simulink model "vehicle_model_2025"  (R2025a)
settings: Solver=ode23tb  StartTime=0.0  StopTime=20  MaxStep=0.001  RelTol=1e-3
model workspace (MAT data in the model file):
  init_r = 0
  init_vx = 0
  init_vy = 0
values from neighbouring files (symbols this model uses):
  Par =     [0_Load_data.mat]
  TireData =     [0_Load_data.mat]
undefined symbols (not defined in the file or in its folder): aero_par, Battery, Motor, SimInput_Steer, SimInput_TorqueFL, SimInput_TorqueFR, SimInput_TorqueRL, SimInput_TorqueRR, sus_par
libraries: simulink x4, BatteryEstimators x1
(part 2 of 2)

== matlab function vehicle_model_2025/Camber/MATLAB Function ==
  data: gamma_FR output; ay input; gamma_FL output; gamma_RL output; gamma_RR output; delta input; Par parameter; sus_par parameter
function [gamma_FR,gamma_FL,gamma_RL,gamma_RR] = fcn(ay,delta,Par, sus_par)

%% Static camber
gamma_static = sus_par.Camber_static;
% track_width = par.TW;
%% SUSPENSION ROLL STIFFNESS
k_phi1 = 10014;  % front axle roll stiffness (Nm/rad)
k_phi2 = 11466;  % rear axle roll stiffness (Nm/rad)

%% ROLL CENTER HEIGHTS
q1 = 0.062;      % front roll center height (m)
q2 = 0.091;      % rear roll center height (m)

%% CAMBER GEOMETRY
b1 = 0.20;       % front IC horizontal distance (m)
b2 = 0.22;       % rear IC horizontal distance (m)

%% TOTAL ROLL STIFFNESS
k_phi_total = k_phi1 + k_phi2;

%% TOTAL VEHICLE ROLL ANGLE
phi = Par.m.*ay.*Par.CG_h / k_phi_total;   % rad

%% AXLE ROLL ANGLES
phi_s1 = phi * (k_phi1 / k_phi_total);   % front suspension roll
phi_s2 = phi * (k_phi2 / k_phi_total);   % rear suspension roll

% Zwc_f = track_width.*0.5.*phi_s1;
% Zwc_r = track_width.*0.5.*phi_s2;
%% CAMBER GAIN COEFFICIENTS
k_gamma_f = - (q1 - b1) / b1;   % front
k_gamma_r = - (q2 - b2) / b2;   % rear

%% Camber due to roll on front axle
delta_gamma_roll_f = k_gamma_f * phi_s1;

%% Camber due to roll on rear axle
delta_gamma_roll_r = k_gamma_r * phi_s2;

%% Camber gain due to heave
% delta_gamma_heave_f = atan(Zwc_f/par.L_fvsa);
% delta_gamma_heave_r = atan(Zwc_r/par.L_fvsa);

%% Camber due to caster 
delta_gamma_caster = atan(tan(sus_par.Caster_static).*sin(delta));

%% Camber angle
gamma_FL = gamma_static + delta_gamma_roll_f + delta_gamma_caster;
gamma_FR = gamma_static - (delta_gamma_roll_f + delta_gamma_caster);
gamma_RL = gamma_static + delta_gamma_roll_r + delta_gamma_caster;
gamma_RR = gamma_static - (delta_gamma_roll_r + delta_gamma_caster);

== matlab function vehicle_model_2025/Simplified Tire Model ==
  data: Fz input; Fx output size=4; slip_ratios input; slip_angles input; camber_angles input; Fy output size=4; Mz output size=4; Mu_x output size=4; Mu_y output size=4; TireData parameter; Par parameter; sus_par parameter
function [Fx, Fy, Mz, Mu_x, Mu_y] = fcn(Fz, slip_ratios, slip_angles, camber_angles, TireData,Par,sus_par)
%#codegen
% =========================================================================
%  VECTORIZED MAGIC FORMULA 5.2 (4-WHEEL)
%  Computes tire physics for all 4 corners simultaneously using element-wise math.
%
%  INPUTS (All 4x1 Vectors):
%    Fz    : Vertical Loads [N] -> [FL; FR; RL; RR]
%    Kappa : Slip Ratios [-]
%    Alpha : Slip Angles [rad]
%    Gamma : Camber Angles [rad]
%    TireData : Parameter Struct (Must be loaded in Base Workspace)
%
%  OUTPUTS (All 4x1 Vectors):
%    Fx    : Longitudinal Force [N]
%    Fy    : Lateral Force [N]
%    Mz    : Self-Aligning Torque [Nm]
%    Mu_x  : Long. Friction Coeff [-]
%    Mu_y  : Lat. Friction Coeff [-]
% =========================================================================

    % 1. EXTRACT PARAMETERS (Scalars)
    p = TireData;
    s = TireData.Scales;
    Fz0 = p.FNOMIN;
    R0  = p.R0;
    par = Par;
    % 2. INPUT SAFETY & NORMALIZATION
    % Clamp negative loads to 0 (Tires can't pull ground)
    Fz_safe = max(Fz, 0); 
    
    % Avoid division by zero for Mu calculations later
    Fz_denom = max(Fz_safe, 1.0); 

    % Normalized Load (dfz) - Vectorized
    dfz = (Fz_safe - Fz0) ./ Fz0;

    % ---------------------------------------------------------------------
    % A. LONGITUDINAL FORCE (Fx) - VECTORIZED
    % ---------------------------------------------------------------------
    Cx = p.PCX1 * s.LCX;
    
    % Friction Coeff Mu_x
    mu_x_base = (p.PDX1 + p.PDX2 .* dfz) .* (1 - p.PDX3 .* camber_angles.^2) .* s.LMUX;
    Dx = mu_x_base .* Fz_safe;
    
    % Stiffness Kx
    Kx = Fz_safe .* (p.PKX1 + p.PKX2 .* dfz) .* exp(p.PKX3 .* dfz) .* s.LKX;
    
    % Stiffness Factor Bx
    Bx = Kx ./ (Cx .* Dx + 1e-6); 
    
    % Shifts (Horizontal & Vertical)
    Shx = (p.PHX1 + p.PHX2 .* dfz) .* s.LHX;
    Svx = Fz_safe .* (p.PVX1 + p.PVX2 .* dfz) .* s.LVX;
    
    % Composite Slip
    k_s = slip_ratios + Shx;
    
    % Curvature Ex (Sign Dependent)
    Ex = (p.PEX1 + p.PEX2 .* dfz + p.PEX3 .* dfz.^2) .* (1 - p.PEX4 .* sign(k_s)) .* s.LEX;
    Ex(Ex > 1) = 1; % Clamp
    
    % Calculation
    Bx_k = Bx .* k_s;
    Fx = Dx .* sin(Cx .* atan(Bx_k - Ex .* (Bx_k - atan(Bx_k)))) + Svx;

    % ---------------------------------------------------------------------
    % B. LATERAL FORCE (Fy) - VECTORIZED
    % ---------------------------------------------------------------------
    Cy = p.PCY1 * s.LCY;
    
    % Friction Coeff Mu_y
    mu_y_base = (p.PDY1 + p.PDY2 .* dfz) .* (1 - p.PDY3 .* camber_angles.^2) .* s.LMUY;
    Dy = mu_y_base .* Fz_safe;
    
    % Cornering Stiffness Ky (Trig Form)
    Ky = p.PKY1 .* Fz0 .* sin(2 .* atan(Fz_safe ./ (p.PKY2 .* Fz0))) .* (1 - p.PKY3 .* abs(camber_angles)) .* s.LKY;
    
    % Poly fallback check (if PKY2 implies poly form)
    if (Ky(1) < 1)
        Ky = Fz_safe .* (p.PKY1 + p.PKY2 .* dfz) .* s.LKY;
    end
    
    By = Ky ./ (Cy .* Dy + 1e-6);
    
    % Shifts
    Shy = (p.PHY1 + p.PHY2 .* dfz) .* s.LHY;
    Svy = Fz_safe .* (p.PVY1 + p.PVY2 .* dfz) .* s.LVY;
    
    a_s = slip_angles + 0*Shy;
    
    % Curvature Ey (Sign Dependent)
    Ey = (p.PEY1 + p.PEY2 .* dfz) .* (1 - (p.PEY3 + p.PEY4 .* camber_angles) .* sign(a_s)) .* s.LEY;
    Ey(Ey > 1) = 1;
    
    % Calculation
    By_a = By .* a_s;
    Fy = -(Dy .* sin(Cy .* atan(By_a - Ey .* (By_a - atan(By_a)))) + 0*Svy);

    % ---------------------------------------------------------------------
    % C. SELF-ALIGNING TORQUE (Mz) - VECTORIZED
    % ---------------------------------------------------------------------
    % Peak Trail Dt
    Dt = (p.QDZ1 + p.QDZ2 .* dfz) .* (1 - p.QDZ3 .* abs(camber_angles)) .* R0 .* s.LTR;
    
    % Trail Slope Bt
    Bt = (p.QBZ1 + p.QBZ2 .* dfz + p.QBZ3 .* dfz.^2) .* (1 + p.QBZ4 .* abs(camber_angles)) .* (s.LKY / s.LMUY);
    
    Ct = p.QCZ1; % Scalar
    Et = (p.QEZ1 + p.QEZ2 .* dfz + p.QEZ3 .* dfz.^2);
    
    % Trail 't' Calculation(Pneumatic trail)
    Bt_a = Bt .* a_s;
    alpha_t = Bt_a - Et .* (Bt_a - atan(Bt_a));
    t = Dt .* cos(Ct .* atan(alpha_t)) .* cos(a_s);

    % Trail 'tm' Calculation(mechanical trail)
    tm = par.R0.*tan(sus_par.Caster_static);

    % Residual Mzr
    Dr = Fz_safe .* R0 .* (p.QDZ6 + p.QDZ7 .* dfz) .* s.LRES;
    Br = 10;
    Mzr = Dr .* cos(atan(Br .* a_s));
    
    % Final Mz (Standard Restoring: Negative Slope)
    % Note: If you want positive slope (sharp tune from before), multiply term by -1.
    Mz = -(t+tm).*Fy + Mzr;

    % ---------------------------------------------------------------------
    % D. OUTPUTS (Zero out lifted wheels)
    % ---------------------------------------------------------------------
    % Friction Coeffs
    Mu_x = Fx ./ Fz_denom;
    Mu_y = Fy ./ Fz_denom;

    % Clean up lifted wheels (Fz <= 0)
    % lifted_idx = Fz <= 0;
    % Fx(lifted_idx) = 0;
    % Fy(lifted_idx) = 0;
    % Mz(lifted_idx) = 0;
    % Mu_x(lifted_idx) = 0;
    % Mu_y(lifted_idx) = 0;

end

== matlab function vehicle_model_2025/roll and pitch angles/theta_constants ==
  data: K_theta output; C_theta output; sus_par parameter; Par parameter
function [K_theta,C_theta] = fcn(sus_par,Par)

% Calculating Pitching stiffness
Kw_fl = sus_par.Ks_f.*(sus_par.Motion_ratio_f)^2; 
Kw_fr = sus_par.Ks_f.*(sus_par.Motion_ratio_f)^2;
Kw_rl = sus_par.Ks_r.*(sus_par.Motion_ratio_r)^2;
Kw_rr = sus_par.Ks_r.*(sus_par.Motion_ratio_r)^2;

K_theta = (Kw_fl + Kw_fr).*(Par.Lf)^2 + (Kw_rl + Kw_rr).*(Par.Lr)^2;

% Calculating Pitch Damping
Cw_fl = sus_par.C_damp_f.*(sus_par.Motion_ratio_f)^2;
Cw_fr = sus_par.C_damp_f.*(sus_par.Motion_ratio_f)^2;
Cw_rl = sus_par.C_damp_r.*(sus_par.Motion_ratio_r)^2;
Cw_rr = sus_par.C_damp_r.*(sus_par.Motion_ratio_r)^2;

C_theta = (Cw_fl + Cw_fr).*(Par.Lf)^2 + (Cw_rl + Cw_rr).*(Par.Lr)^2;

% Kw = [Kw_fl;Kw_fr;Kw_rl;Kw_rr];

== matlab function vehicle_model_2025/roll and pitch angles/Phi_constants ==
  data: K_phi output; C_phi output; Par parameter; sus_par parameter
function [K_phi,C_phi] = fcn(Par, sus_par)

% Calculating Pitching stiffness
Kw_fl = sus_par.Ks_f.*(sus_par.Motion_ratio_f)^2; 
Kw_fr = sus_par.Ks_f.*(sus_par.Motion_ratio_f)^2;
Kw_rl = sus_par.Ks_r.*(sus_par.Motion_ratio_r)^2;
Kw_rr = sus_par.Ks_r.*(sus_par.Motion_ratio_r)^2;

K_phi = (Kw_fl + Kw_fr).*(Par.TW/2)^2 + (Kw_rl + Kw_rr).*(Par.TW/2)^2;

% Calculating Pitch Damping
Cw_fl = sus_par.C_damp_f.*(sus_par.Motion_ratio_f)^2;
Cw_fr = sus_par.C_damp_f.*(sus_par.Motion_ratio_f)^2;
Cw_rl = sus_par.C_damp_r.*(sus_par.Motion_ratio_r)^2;
Cw_rr = sus_par.C_damp_r.*(sus_par.Motion_ratio_r)^2;

C_phi = (Cw_fl + Cw_fr).*(Par.TW/2)^2 + (Cw_rl + Cw_rr).*(Par.TW/2)^2;

== matlab function vehicle_model_2025/Battery Pack/MATLAB Function ==
  data: Voc_pack input; v_bus output; R0_pack input; V_rc input; I_dc input
function v_bus = fcn(Voc_pack, R0_pack, V_rc, I_dc)
    % This function calculates the terminal voltage of the battery pack.
    % Voc_pack: Output from OCV LUT multiplied by Ns
    % R0_pack:  Output from R0 LUT multiplied by (Ns/Np)
    % V_rc:     Instantaneous voltage across the RC branch
    % I_dc:     Total DC current from the motor

    % 1. Calculate the instantaneous Ohmic drop (Ohm's Law)
    V_ohmic = I_dc * R0_pack;

    % 2. Calculate terminal voltage (Vt = Voc - V_ohmic - V_rc)
    v_bus = Voc_pack - V_ohmic - V_rc;

    % 3. Safety: Ensure voltage doesn't drop below a physical floor (e.g., 2.5V * Ns)
    % This prevents simulation crashes if the battery is fully depleted.
    v_bus = max(v_bus, 2.5 * 144); 
end

== matlab function vehicle_model_2025/Brakes/MATLAB Function ==
  data: brake_pedal input; T_brakes output; omega input; Brake parameter
function T_brakes = fcn(brake_pedal, omega, Brake)
    % BRAKE TORQUE CALCULATION
    % Converts normalized pedal/actuator position into physical torque
    % and ensures torque direction opposes wheel rotation.
    
    % 1. Calculate Magnitude of Torque based on Command (0-1)
    % We use the static max targets from the design sheet
    T_mag_Front = brake_pedal * Brake.MaxTorque_Wheel_F;
    T_mag_Rear  = brake_pedal * Brake.MaxTorque_Wheel_R;
    
    % Initialize output vector (FL, FR, RL, RR)
    T_brakes = zeros(4, 1);
    
    % 2. Apply Torque per Wheel with Directional Logic
    % Loop through all 4 wheels to apply logic individually
    % Indices: 1=FL, 2=FR, 3=RL, 4=RR
    
    for i = 1:4
        % Determine if this is a Front (1,2) or Rear (3,4) wheel
        if i <= 2
            T_req = T_mag_Front;
        else
            T_req = T_mag_Rear;
        end
        
        % Directional Check:
        % Torque must be negative if omega is positive, and vice versa.
        % -sign(omega) flips the torque direction.
        T_applied = T_req * -sign(omega(i));
        
        % Zero-Speed Cutoff:
        % If wheel is nearly stopped, clamp torque to zero to prevent 
        % the simulation from "driving" the car backwards.
        if abs(omega(i)) < Brake.ZeroSpeedThreshold
            T_applied = 0;
            
            % Advanced: Ideally, below threshold, T_brake should act as 
            % a viscous damper or Coulomb friction that exactly cancels 
            % remaining motion, but zeroing is sufficient for laptime sims.
        end
        
        T_brakes(i) = T_applied;
    end
end

== matlab function vehicle_model_2025/Motor/MATLAB Function ==
  data: rpm input; Torque_Nm output; throttle input; v_dc input
function Torque_Nm = fcn(rpm, throttle, v_dc)
    % 1. Constants
    p = 4;                      % Pole pairs 
    L = 0.393e-3;               % Inductance
    kt = 0.492;
    psi_m = kt/(1.5*p*sqrt(2));              % Flux linkage derived from kt
    I_lim = 61; % Peak phase current 
    V_max = v_dc / sqrt(3);     % Maximum available phase voltage
    
    % 2. Speed Conversion
    omega_m = rpm * (2*pi/60);
    omega_e = p * omega_m;
    
    % 3. MTPA / Field Weakening Logic
    if omega_e < 1e-3 % Handle standstill
        iq = I_lim* sqrt(2) * throttle;
        id = 0;
    else
        % Calculate required voltage for MTPA (id=0)
        V_req = omega_e * sqrt((L*I_lim)^2 + psi_m^2);
        
        if V_req <= V_max
            % Below base speed
            iq = I_lim;
            id = 0;
        else
            % Above base speed (Field Weakening)
            % Solving the quadratic for iq at the boundary of V_max and I_lim
            a = (omega_e * L)^2;
            b = 2 * omega_e^2 * L * psi_m;
            c = (omega_e * psi_m)^2 + (omega_e * L * I_lim)^2 - V_max^2;
            
            % Simple analytical approximation for constant power region
            iq = min(I_lim, V_max / (omega_e * L));
        end
    end
    
    % 4. Final Torque Calculation (with 29.1 Nm cap)
    Torque_Nm = min(29.1, 1.5 * p * psi_m * iq / sqrt(2)); 
end

== matlab function vehicle_model_2025/Motor/MATLAB Function1 ==
  data: rpm_feedback input; Torque_Nm output; throttle input; v_dc_bus input
function Torque_Nm = fcn(rpm_feedback, throttle, v_dc_bus)
    % --- 1. Define Motor Constants from Datasheet ---
    p = 4;                          % Number of pole pairs 
    L = 0.393e-3;                   % Phase inductance in Henries 
    kt = 0.492;                     % Torque constant in Nm/Arms 
    psi_m = kt / (1.5 * p * sqrt(2)); % Calculate magnet flux linkage (~0.058 Wb)
    I_max_rms = 61;                 % Maximum peak current in Arms 
    n_max = 20000;                  % Maximum mechanical RPM limit 
    T_peak_limit = 29.1;            % Absolute peak torque cap in Nm 

    % --- 2. Enforce Hard Mechanical RPM Limit ---
    if abs(rpm_feedback) >= n_max   % Check if current speed exceeds mechanical redline
        Torque_Nm = 0;              % Kill all torque production at the limit
        return;                     % Exit function immediately
    end

    % --- 3. Convert Inputs to Electrical Units ---
    omega_m = rpm_feedback * (2*pi/60);      % Convert mechanical RPM to rad/s
    omega_e = omega_m * p;                   % Convert mechanical speed to electrical frequency
    V_max_phase = v_dc_bus / sqrt(3);        % Calculate max phase voltage (fundamental limit)
    I_cmd_peak = I_max_rms * sqrt(2) * throttle; % Scaled peak current command based on throttle

    % --- 4. Determine Operating Region (MTPA vs. Field Weakening) ---
    % Calculate the voltage required for MTPA (where id = 0)
    % Equation: V = omega_e * sqrt( (L*iq)^2 + (psi_m)^2 )
    V_required_mtpa = abs(omega_e) * sqrt((L * I_cmd_peak)^2 + psi_m^2);

    if V_required_mtpa <= V_max_phase        % If enough voltage is available for requested torque
        % REGION 1: Below Base Speed (Maximum Torque Per Ampere)
        id = 0;                              % No d-axis current needed (standard operation)
        iq = I_cmd_peak;                     % All available current used for torque production
    else
        % REGION 2: Above Base Speed (Field Weakening)
        % We must inject negative d-axis current (id) to oppose psi_m and stay within V_max
        % Intersection of Current Circle (id^2 + iq^2 = I^2) and Voltage Ellipse
        
        % Solving the voltage ellipse for id:
        % (V_max/omega_e)^2 = (L*iq)^2 + (L*id + psi_m)^2
        % This simplifies to a quadratic equation for id
        a_quad = L^2;                        % Quadratic coefficient 'a'
        b_quad = 2 * L * psi_m;              % Quadratic coefficient 'b'
        c_quad = psi_m^2 + (L * I_cmd_peak)^2 - (V_max_phase / omega_e)^2; % Coefficient 'c'
        
        % Calculate the required negative d-axis current using the quadratic formula
        id = (-b_quad + sqrt(b_quad^2 - 4 * a_quad * c_quad)) / (2 * a_quad);
        
        % Enforce physical bounds on current components
        id = max(min(id, 0), -I_cmd_peak);   % Clamp id between -I_max and 0
        iq = sqrt(max(0, I_cmd_peak^2 - id^2)); % Solve for remaining q-axis current
    end

    % --- 5. Calculate Final Torque Output ---
    % Standard PMSM Torque Equation: Te = 1.5 * p * psi_m * iq
    T_generated = 1.5 * p * psi_m * iq;      % Calculate the raw electromagnetic torque
    
    % Final output is capped by the mechanical peak torque of the motor
    Torque_Nm = min(T_generated, T_peak_limit); % Saturate at 29.1 Nm 
end

== matlab function vehicle_model_2025/Motor/Motor with Field Weakening ==
  data: rpm_4x1 input; Torque_Nm_vec output; throttle_scalar input; v_dc_bus input; Motor parameter; I_dc_total output size=[1]; P_total_sum output size=[1]
function [Torque_Nm_vec, I_dc_total,P_total_sum] = fcn(rpm_4x1, throttle_scalar, v_dc_bus, Motor)
    % Inputs:
    %   rpm_4x1         : [FL; FR; RL; RR] wheel speeds in RPM
    %   throttle_scalar : Driver input (0 to 1)
    %   v_dc_bus        : Battery voltage (V)
    %   Motor           : Struct containing constants
    
    % --- 1. Distribute Inputs ---
    % We apply the same throttle to both motors for now.
    % We extract the Rear-Left (index 3) and Rear-Right (index 4) speeds.
    rpm_targets = [rpm_4x1(3); rpm_4x1(4)]; 
    throttle_vec = [throttle_scalar; throttle_scalar];

    % Initialize storage
    Torque_Nm_vec = zeros(2, 1); % [T_RL; T_RR]
    P_elec_vec = zeros(2, 1);
    
    for i = 1:2
        % --- 2. Redline & Mechanical Limit Check ---
        if abs(rpm_targets(i)) >= Motor.n_max
            continue; % Torque and Power remain 0
        end

        % --- 3. Electrical Conversions ---
        omega_m = rpm_targets(i) * (2*pi/60);
        omega_e = max(abs(omega_m * Motor.p), 0.1); 
        V_max_phase = v_dc_bus / sqrt(3);
        I_cmd_peak = Motor.I_max_rms * sqrt(2) * throttle_vec(i);

        % --- 4. Region Selection: MTPA vs Field Weakening ---
        V_req_mtpa = omega_e * sqrt((Motor.L * I_cmd_peak)^2 + Motor.psi_m^2);
        
        if V_req_mtpa <= V_max_phase
            id = 0;
            iq = I_cmd_peak;
        else
            % Field Weakening logic for Fischer Motor
            a = Motor.L^2;
            b = 2 * Motor.L * Motor.psi_m;
            c = Motor.psi_m^2 + (Motor.L * I_cmd_peak)^2 - (V_max_phase / omega_e)^2;
            
            id = (-b + sqrt(max(0, b^2 - 4 * a * c))) / (2 * a);
            id = max(min(id, 0), -I_cmd_peak); 
            iq = sqrt(max(0, I_cmd_peak^2 - id^2));
        end

        % --- 5. Torque and Power Calculation ---
        T_gen = 1.5 * Motor.p * Motor.psi_m * iq;
        Torque_Nm_vec(i) = min(T_gen, Motor.T_peak_limit);

        % P_elec = P_mechanical + P_copper_losses
        P_mech = abs(Torque_Nm_vec(i) * omega_m);
        P_copper = 3 * 0.126 * (I_cmd_peak / sqrt(2))^2;
        P_elec_vec(i) = P_mech + P_copper;
    end

    % --- 6. Battery Summation ---
    P_total_sum = sum(P_elec_vec);
    if v_dc_bus > 20
        % Calculate total current draw for the Molicel P45B pack
        I_dc_total = P_total_sum / (0.95 * v_dc_bus);

    else
        I_dc_total = 0;
    end
end

== matlab function vehicle_model_2025/Torque Distribution/MATLAB Function ==
  data: T_motor input; omega input; T_FL output; T_brake_vec input; T_FR output; T_RL output; T_RR output
function [T_FL, T_FR, T_RL, T_RR] = torque_combiner(T_motor, omega, T_brake_vec)
    % INPUTS:
    % T_motor:     2x1 [Left, Right] Motor Torque Request (from Throttle)
    % omega:       4x1 [FL, FR, RL, RR] Wheel Speeds (rad/s)
    % T_brake_vec: 4x1 Brake Capacity (Negative values expected)

    % --- 1. INITIALIZATION ---
    T_FL = 0.0; T_FR = 0.0; T_RL = 0.0; T_RR = 0.0;
    
    % PARAMETERS
    w_threshold = 2.0;  % [rad/s] Speed below which we switch to linear damping
    brake_active_threshold = 100.0; % [Nm] Torque to consider "Brakes Active"

    % Get absolute brake capacities
    B_FL = abs(T_brake_vec(1));
    B_FR = abs(T_brake_vec(2));
    B_RL = abs(T_brake_vec(3));
    B_RR = abs(T_brake_vec(4));

    % --- 2. BRAKE PRIORITY LOGIC (The Fix for Rear Spin) ---
    % If the driver is braking hard, we CUT or REDUCE motor torque.
    % This prevents the "fighting" that causes the rear wheels to spin at 115 rad/s.
    
    total_brake_force = B_FL + B_FR + B_RL + B_RR;
    
    % Factor: 1.0 = Full Drive, 0.0 = Throttle Cut
    % If braking > threshold, we smoothly cut throttle to 0.
    if total_brake_force > brake_active_threshold
        throttle_factor = 0.0; 
    else
        throttle_factor = 1.0;
    end
    
    % Apply the cut to the motor inputs
    T_motor_effective = T_motor * throttle_factor;


    % --- 3. ROBUST BRAKE CALCULATION (Viscous Region) ---
    % This local logic prevents solver crashes when wheels lock (w=0)
    % It uses linear damping near zero speed.
    
    % Fronts (Brake Only)
    T_FL = apply_brake_physics(omega(1), B_FL, w_threshold);
    T_FR = apply_brake_physics(omega(2), B_FR, w_threshold);

    % Rears (Motor + Brake)
    T_brake_RL = apply_brake_physics(omega(3), B_RL, w_threshold);
    T_brake_RR = apply_brake_physics(omega(4), B_RR, w_threshold);
    
    % Combine: Effective Motor (Positive) + Braking (Negative)
    T_RL = T_motor_effective(1) + T_brake_RL;
    T_RR = T_motor_effective(2) + T_brake_RR;
end

% --- HELPER LOGIC ---
function T_out = apply_brake_physics(w, Capacity, w_th)
    % If moving fast: Constant Friction (Capacity)
    % If moving slow: Viscous Damping (Linear line to 0)
    if abs(w) < w_th
        % Linear region (Like moving through honey)
        % This forces the torque to exactly 0 as speed hits 0.
        T_out = -Capacity * (w / w_th);
    else
        % Sliding region (Full friction)
        T_out = -Capacity * sign(w);
    end
end

== matlab function vehicle_model_2025/Normal_loads/ARB/MATLAB Function ==
  data: Zs input; F_arb output; sus_par parameter
function F_arb = fcn(Zs,sus_par)

  % Calculation of Anti roll bar forces at each wheel
    delta_zf = Zs(1) - Zs(2);
    delta_zr = Zs(3) - Zs(4);

    F_arb_fl = sus_par.K_arb_f*delta_zf/2;
    F_arb_fr = -sus_par.K_arb_f*delta_zf/2;
    F_arb_rl = sus_par.K_arb_r*delta_zr/2;
    F_arb_rr = -sus_par.K_arb_r*delta_zr/2;

    F_arb = [F_arb_fl ; F_arb_fr ; F_arb_rl ; F_arb_rr];

== matlab function vehicle_model_2025/Normal_loads/MATLAB Function ==
  data: F_arb input; F_spring input; Fz output; Par parameter
function Fz = fcn(F_arb , F_spring,Par)
m_us = [12;12;18;18];
g = Par.g;
F_unsprung = m_us.*g;
Fz = F_unsprung - (F_spring + F_arb);

== matlab function vehicle_model_2025/Visualise slip_ratios/MATLAB Function ==
  data: kappa input; K_fl output; K_fr output; K_rl output; K_rr output
function [K_fl,K_fr,K_rl,K_rr] = fcn(kappa)

K_fl = kappa(1);

K_fr = kappa(2);

K_rl = kappa(3);

K_rr = kappa(4);

end

== matlab function vehicle_model_2025/Visualise slip_angles/MATLAB Function ==
  data: slip_angles input; alpha_fl output; alpha_fr output; alpha_rl output; alpha_rr output
function [alpha_fl,alpha_fr,alpha_rl,alpha_rr] = fcn(slip_angles)

alpha_fl = slip_angles(1);

alpha_fr = slip_angles(2);

alpha_rl = slip_angles(3);

alpha_rr = slip_angles(4);

end

== matlab function vehicle_model_2025/Visualise_Fx_tire/MATLAB Function ==
  data: Fx_tire input; Fx_fl output; Fx_fr output; Fx_rl output; Fx_rr output
function [Fx_fl,Fx_fr,Fx_rl,Fx_rr]  = fcn(Fx_tire)

Fx_fl = Fx_tire(1);

Fx_fr = Fx_tire(2);

Fx_rl = Fx_tire(3);

Fx_rr = Fx_tire(4);

end

== matlab function vehicle_model_2025/Visualise_Fy_tire/MATLAB Function ==
  data: Fy_tire input; Fy_fl output; Fy_fr output; Fy_rl output; Fy_rr output
function [Fy_fl,Fy_fr,Fy_rl,Fy_rr]  = fcn(Fy_tire)

Fy_fl = Fy_tire(1);

Fy_fr = Fy_tire(2);

Fy_rl = Fy_tire(3);

Fy_rr = Fy_tire(4);

end

== matlab function vehicle_model_2025/Visualise_Fx_tire1/MATLAB Function ==
  data: Fz_tire input; Fz_fl output; Fz_fr output; Fz_rl output; Fz_rr output
function [Fz_fl,Fz_fr,Fz_rl,Fz_rr]  = fcn(Fz_tire)

Fz_fl = Fz_tire(1);

Fz_fr = Fz_tire(2);

Fz_rl = Fz_tire(3);

Fz_rr = Fz_tire(4);

end

== matlab function vehicle_model_2025/Normal_loads/MATLAB Function1 ==
  data: v input; F_aero_down output; aero_par parameter
function F_aero_down = fcn(v,aero_par)

% Aerodynamic constants:
rho = aero_par.rho;
area = aero_par.Area;
Cl = aero_par.Cl;

F_aero_down = -0.5*rho*Cl*area*(v^2);

== matlab function vehicle_model_2025/Normal_loads/Spring_forces/MATLAB Function ==
  data: theta input; phi input; F_aero_total input; Zs output; F_spring output; Par parameter; aero_par parameter; sus_par parameter
function [Zs,F_spring] = fcn(theta, phi, F_aero_total, Par, aero_par, sus_par)

  % 1. Constants
    g = Par.g;
    L = Par.WB;    % Wheelbase
    T = Par.TW;
    h = Par.CG_h;  % CG Height
    m = Par.m;
    ms = Par.sprung_mass;
    mus = Par.unsprung_mass;
    half_T = T/2;
   

    % Calculating Pitching stiffness
    Kw_fl = sus_par.Ks_f.*(sus_par.Motion_ratio_f)^2; 
    Kw_fr = sus_par.Ks_f.*(sus_par.Motion_ratio_f)^2;
    Kw_rl = sus_par.Ks_r.*(sus_par.Motion_ratio_r)^2;
    Kw_rr = sus_par.Ks_r.*(sus_par.Motion_ratio_r)^2;

    Kw = [Kw_fl;Kw_fr;Kw_rl;Kw_rr];

    % Front and rear Wheelbase
    Lf = L*0.51;  % Front wheel base
    Lr = L*0.49;  % Rear wheel base

    % Static load due to sprung mass and unsprung mass at each wheel
    F_sprung_mass = ms*g/4;
    F_unsprung_mass = mus.*g;

    % Stiffness at each wheel:
    Kt = 90000;
    stiff_1 = Kw(1)*Kt/(Kw(1)+Kt);
    stiff_2 = Kw(2)*Kt/(Kw(2)+Kt);
    stiff_3 = Kw(3)*Kt/(Kw(3)+Kt);
    stiff_4 = Kw(4)*Kt/(Kw(4)+Kt);
    
    % Vertical deflection of each suspension(compression = -ve)
    zsfl = -(F_sprung_mass)/stiff_1 + Lf*theta + (T/2)*phi - 0.5 * F_aero_total * (1 - aero_par.CP_rear)/stiff_1;
    zsfr = -(F_sprung_mass)/stiff_2 + Lf*theta - (T/2)*phi - 0.5 * F_aero_total * (1 - aero_par.CP_rear)/stiff_2;
    zsrl = -(F_sprung_mass)/stiff_3 - Lr*theta + (T/2)*phi - 0.5 * F_aero_total*(aero_par.CP_rear)/stiff_3;
    zsrr = -(F_sprung_mass)/stiff_4 - Lr*theta - (T/2)*phi - 0.5 * F_aero_total*(aero_par.CP_rear)/stiff_4;

    Zs = [zsfl;zsfr;zsrl;zsrr];

    % Spring force at each wheel
    Fs_fl = stiff_1*zsfl;
    Fs_fr = stiff_2*zsfr;
    Fs_rl = stiff_3*zsrl;
    Fs_rr = stiff_4*zsrr;

    F_spring = [Fs_fl;Fs_fr;Fs_rl;Fs_rr];

== matlab function vehicle_model_2025/slip ratios ==
  data: Vx input; Vy input; slip_ratios output; yawrate input; Omega input; Steer_FL input; Steer_FR input; Par parameter
function slip_ratios = fcn(Vx,Vy, yawrate, Omega,Steer_FL,Steer_FR, Par)
%#codegen


    % 1. Constants
    T = Par.TW;
    Re = Par.R0;
    half_T = T / 2;
    a= Par.Lf;
    b=Par.Lr;
    r = yawrate;
    % 2 Yaw Rate Correction (Kinematics)
    
    Vx_FL = Vx - yawrate * half_T;  % Left
    Vx_FR = Vx + yawrate * half_T;  % Right
    Vx_RL = Vx - yawrate * half_T;
    Vx_RR = Vx + yawrate * half_T;
    
    Vx_vec = [Vx_FL; Vx_FR; Vx_RL; Vx_RR];
    
    Vy_FL = Vy + r * a;
    Vy_FR = Vy+ r * a;
    Vy_RL = Vy- r * b;
    Vy_RR = Vy- r * b;

    Vy_vec = [Vy_FL; Vy_FR; Vy_RL; Vy_RR];
    Delta = [Steer_FL;Steer_FR;0;0];
    % 3. Slip Angle Correction (Projection)
 
    V_road_plane = Vx_vec .* cos(Delta) + Vy_vec .* sin(Delta);

    % 4. Calculate Wheel Linear Speed
    V_wheel = Omega .* Re;

    % 5. Calculate Slip Ratio
    V_safe_threshold = 0.1; 
    V_ref = max(abs(V_road_plane), V_safe_threshold);
    
    slip_ratios_raw = (V_wheel - V_road_plane) ./ V_ref;
    slip_ratios = min(max(slip_ratios_raw,-1),1);
end

== matlab function vehicle_model_2025/Normal_loads/Visualise sus disp/MATLAB Function ==
  data: Zs input; zsfl output; zsfr output; zsrl output; zsrr output
function [zsfl,zsfr,zsrl,zsrr] = fcn(Zs)

zsfl = Zs(1);
zsfr = Zs(2);
zsrl = Zs(3);
zsrr = Zs(4);

end

== matlab function vehicle_model_2025/Slip Angles ==
  data: Vx input; slip_angles output; Vy input; yawrate input; Steer_FL input; Steer_FR input; Par parameter
function slip_angles = fcn(Vx, Vy, yawrate, Steer_FL, Steer_FR, Par)
%#codegen

    % 1. Geometry Setup
    L = Par.WB;
    T = Par.TW;
    
    % Distance from CG to Axles
    a = L * Par.WD_r;     
    b = L - a;             
    half_T = T / 2;

    % 2. Calculate Velocity Components at Each Corner
    % Kinematic transformation from CG to Hubs
    % Front Left (1)
        Vx_FL = Vx - yawrate * half_T;
        Vy_FL = Vy + yawrate * a;
    
    % Front Right (2)
        Vx_FR = Vx + yawrate * half_T;
        Vy_FR = Vy + yawrate * a;
    
    % Rear Left (3)
        Vx_RL = Vx - yawrate * half_T;
        Vy_RL = Vy - yawrate * b;
    
    % Rear Right (4)
        Vx_RR = Vx + yawrate * half_T;
        Vy_RR = Vy - yawrate * b;

    % 3. Calculate Velocity Angles (Theta_V)

        Theta_FL = atan2(Vy_FL, max(Vx_FL,0.1)); 
        Theta_FR = atan2(Vy_FR, max(Vx_FR,0.1));
        Theta_RL = atan2(Vy_RL, max(Vx_RL,0.1));
        Theta_RR = atan2(Vy_RR, max(Vx_RR,0.1));
    
    % 4. Construct Steering Vector (Delta)
    % Rears are assumed fixed (0 steering)
        Delta = [Steer_FL; Steer_FR; 0; 0];
    
    % Vector of Velocity Angles
        Theta_V = [Theta_FL; Theta_FR; Theta_RL; Theta_RR];

    % 5. Final Calculation
    % Alpha = Delta - Theta_V
        slip_angles = Delta - Theta_V ;
end

== matlab function vehicle_model_2025/Wheel to Vehicle Coordinates ==
  data: Fx_w input; Fx_b output; Fy_w input; Steer_FL input; Steer_FR input; Fy_b output
function [Fx_b, Fy_b] = fcn(Fx_w, Fy_w, Steer_FL, Steer_FR)
%#codegen
% FORCE & MOMENT RESOLVER
    % 1. Construct Steering Vector [FL; FR; RL; RR]
    % Rear steering is assumed to be 0
    Delta = [Steer_FL; Steer_FR; 0; 0];
    
    % 2. Pre-calculate Trig functions (Vectorized)
    c_d = cos(Delta);
    s_d = sin(Delta);
    
    % Longitudinal Body Force:

    Fx_b = Fx_w .* c_d - Fy_w .* s_d;
    
    % Lateral Body Force:
    % Fy_body = Fx_wheel * sin(delta) + Fy_wheel * cos(delta)
    Fy_b = Fx_w .* s_d + Fy_w .* c_d;
    
    % 4. Summation: Total Forces acting on CG
    %B_Fx = sum(Fx_b);
    %B_Fy = sum(Fy_b);
    
end

== matlab function vehicle_model_2025/Steering Kinematics/Steering Kinematics ==
  data: Steer_Input input; Ackermann_Pct input; Steer_FL output; Steer_FR output; Par parameter
function [Steer_FL, Steer_FR] = fcn(Steer_Input, Ackermann_Pct, Par)
%#codegen

    % 1. Constants
    L = Par.WB;      % Wheelbase
    half_T = Par.TW / 2; % Half Track Width

    % 2. Safety Clamp (Prevent tan(90) singularity)
    delta = min(max(Steer_Input, -1.5), 1.5); 
    
    % 3. Calculate "Pure Ackermann" Angles
    % Ideally, inner wheel turns sharper than outer wheel.
    tan_d = tan(delta);
    
    % FL (Left): Denom depends on sign of turn.
    % If turning Left (+), Denom shrinks (Sharper).
    FL_Ack = atan( (L * tan_d) / (L - half_T * tan_d) );
    
    % FR (Right): 
    % If turning Left (+), Denom grows (Shallower).
    FR_Ack = atan( (L * tan_d) / (L + half_T * tan_d) );
    
    % 4. Calculate "Parallel" Angles
    % Both wheels exactly match the center input
    FL_Par = delta;
    FR_Par = delta;
    
    % 5. Linear Blend based on Percentage
    % Formula: Final = Parallel + (Ackermann - Parallel) * Percent
    Steer_FL = FL_Par + (FL_Ack - FL_Par) * Ackermann_Pct;
    Steer_FR = FR_Par + (FR_Ack - FR_Par) * Ackermann_Pct;

end

== matlab function vehicle_model_2025/Wheel Dynamics/MATLAB Function ==
  data: T_in input; Omega_dot output; Fx_rr input; Fx_tire input; Omega input; Par parameter
function Omega_dot = fcn(T_in, Fx_rr,Fx_tire, Omega, Par)
%#codegen

    % 1. Constants
    R = Par.R0;
    Iw = Par.Iw;

    % 2. Separate Drive and Brake components

    T_drive = max(T_in, 0); 
    
    % T_brake is the magnitude of the negative part of T_in
    T_brake_mag = abs(min(T_in, 0));
    

    Rotation_Dir = tanh(10 * Omega);

    % 4. Calculate Net Torque
    T_tire_reaction = abs(Fx_rr .* R);
    T_tire = Fx_tire .*R;
    T_damping = 0.1*Omega;
    T_net = T_drive - (T_brake_mag .* Rotation_Dir) - (T_tire_reaction.*Rotation_Dir) -T_tire - T_damping;

    % 5. Compute Angular Acceleration
    Omega_dot = T_net ./ Iw;

end

== matlab function vehicle_model_2025/Rolling Resistance ==
  data: Fz input; wFx_rr output; Omega input; slip_angles input; Par parameter
function wFx_rr  = fcn(Fz, Omega,slip_angles, Par)
%#codegen

    % 1. Calculate Total Magnitude
    F_mag = Par.C_rr .* abs(Fz);

    % 2. Determine Direction
    Dir = tanh(10 * Omega);

    
    % X-Component: Resists Spin (Torque generating)
    % wFx = -Magnitude * Direction * cos(Alpha)
    wFx_rr = -F_mag .*Dir.* cos(slip_angles);

end
